simulink model "test_mpu6050"  (R2024b)
settings: Solver=FixedStepAuto  StartTime=0.0  StopTime=60  FixedStep=dt  RelTol=1e-3
model workspace (MAT data in the model file):
  dt = Simulink.Parameter
  dt.Value = 0.001
  dt.Complexity = 'real'
  dt.Dimensions = [1 1]
  dt.DataType = 'auto'
libraries: simulink x2
settings Model: ExtModeTrigDuration=2  Creator=schwmaxi  LastModifiedBy=schwmaxi
settings SolverCC: PositivePriorityOrder=on
settings OptimizationCC: BlockReduction=off  BooleanDataType=off  DefaultParameterBehavior=Inlined  EnhancedBackFolding=on  PassReuseOutputArgsAs=Individual arguments  ZeroExternalMemoryAtStartup=off  ZeroInternalMemoryAtStartup=off  MaxStackSize=200000  OptimizeBlockOrder=speed  DifferentSizesBufferReuse=on  OptimizationCustomize=off  EfficientTunableParamExpr=on
settings DebuggingCC: SaveWithParameterizedLinksMsg=none  UnderspecifiedInitializationDetection=Classic  MergeDetectMultiDrivingBlocksExec=none  SignalResolutionControl=TryResolveAllWithWarning  ParameterTunabilityLossMsg=error
settings HardwareCC: ProdBitPerPointer=32  ProdBitPerSizeT=32  ProdBitPerPtrDiffT=32  ProdLargestAtomicInteger=Long  ProdLargestAtomicFloat=Double  ProdWordSize=32  ProdLongLongMode=on  ProdHWDeviceType=ARM Compatible->ARM Cortex-A (32-bit)  UseEmbeddedCoderFeatures=off
settings ModelReferenceCC: PropagateSignalLabelsOutOfModel=off
settings RTWCC: Description=Embedded Coder  SystemTargetFile=ert.tlc  HardwareBoard=Raspberry Pi  TLCOptions="-aInlineSetEventsForThisBaseRateFcn=TLC_FALSE -aSuppressMultiTaskScheduler=TLC_FALSE  -aRateBasedStepFcn=0"  TemplateMakefile=ert_default_tmf  Toolchain=GNU GCC Embedded Linux
settings CodeAppCC: ForceParamTrailComments=on  IgnoreCustomStorageClasses=off  OperatorAnnotations=on  SimulinkDataObjDesc=on  SFDataObjDesc=on  InsertBlockDesc=on
settings ERTTargetCC: SupportNonInlinedSFcns=on  SupportVariableSizeSignals=on  ExtModeTransport=2  ExtModeStaticAlloc=on  ExtModeMexFile=ext_xcp  ExtModeIntrfLevel=Level2 - Open

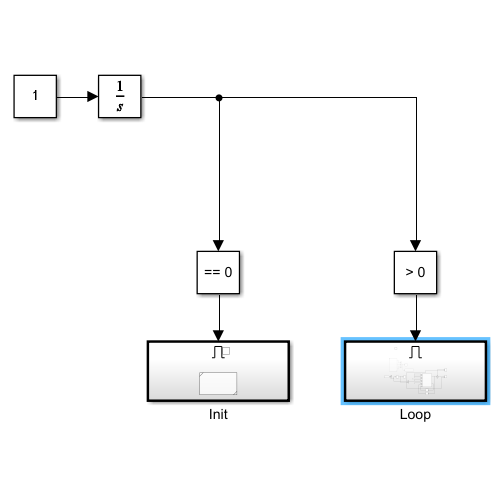
[thumbnail: Simulink's stored preview of the top-level diagram]
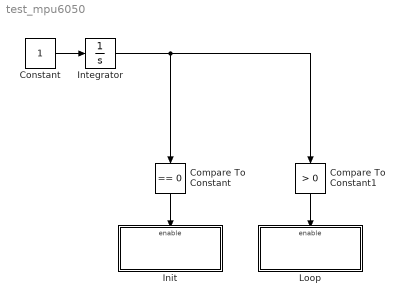
== system test_mpu6050 ==
  Compare To Constant : simulink/Logic and Bit Operations/Compare To Constant  relop===  const=0  OutDataTypeStr=boolean
  Compare To Constant1 : simulink/Logic and Bit Operations/Compare To Constant  relop=>  const=0  OutDataTypeStr=boolean
  Constant : Constant
  Init : Subsystem  TreatAsAtomicUnit=on
  Integrator : Integrator
  Loop : Subsystem  TreatAsAtomicUnit=on
  wires:
  Compare To Constant/1 -> Init/Enable
  Integrator/1 -> Compare To Constant1/1, Compare To Constant/1
  Constant/1 -> Integrator/1
  Compare To Constant1/1 -> Loop/Enable

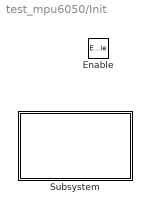
== system test_mpu6050/Init ==
  Enable : EnablePort
  Subsystem : Subsystem  ReferencedSubsystem=InitIMU

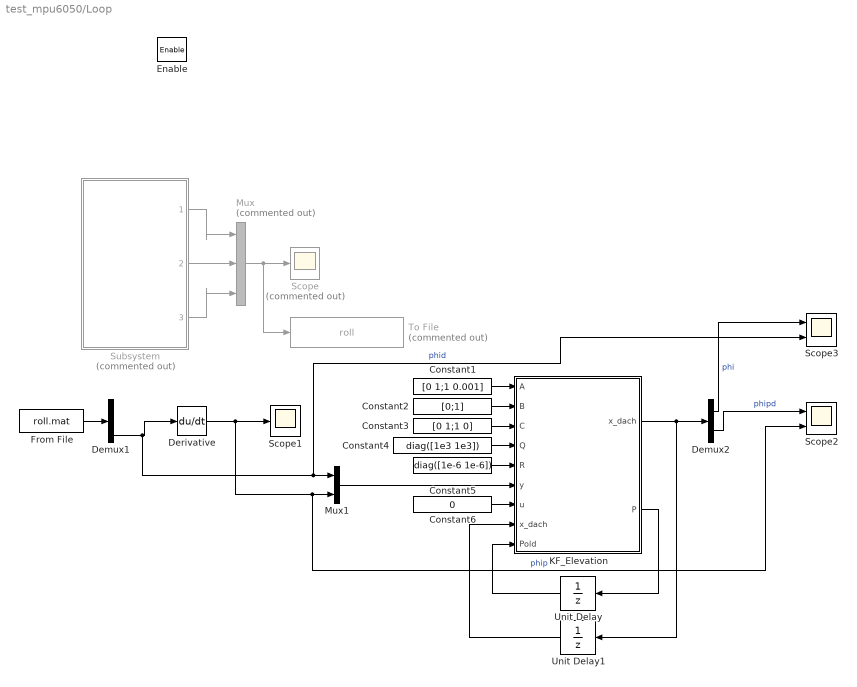
== system test_mpu6050/Loop ==
  Enable : EnablePort
  Constant1 : Constant  Value=[0 1;1 0.001]  VectorParams1D=off
  Constant2 : Constant  Value=[0;1]  VectorParams1D=off
  Constant3 : Constant  Value=[0 1;1 0]  VectorParams1D=off
  Constant4 : Constant  Value=diag([1e3 1e3])  VectorParams1D=off
  Constant5 : Constant  Value=diag([1e-6 1e-6])  VectorParams1D=off
  Constant6 : Constant  Value=0  VectorParams1D=off
  Demux1 : Demux  Outputs=3
  Demux2 : Demux  Outputs=2
  Derivative : Derivative
  From File : FromFile  FileName=roll.mat  SampleTime=0
  KF_Elevation : MATLAB Function  TreatAsAtomicUnit=on
  Mux : Mux  Commented=on  Inputs=3
  Mux1 : Mux  Inputs=2
  Scope : Scope  Commented=on
  Scope1 : Scope
  Scope2 : Scope  NumInputPorts=2
  Scope3 : Scope  NumInputPorts=2
  Subsystem : Subsystem  Commented=on  ReferencedSubsystem=IMU
  To File : ToFile  Commented=on  Filename=roll  SampleTime=0.001
  Unit Delay : UnitDelay  InitialCondition=diag([1 1e10])  SampleTime=-1  HasFrameUpgradeWarning=on
  Unit Delay1 : UnitDelay  InitialCondition=zeros(2,1)  SampleTime=-1  HasFrameUpgradeWarning=on
  wires:
  Subsystem/2 -> Mux/2
  Subsystem/1 -> Mux/1
  Subsystem/3 -> Mux/3
  Mux/1 -> To File/1, Scope/1
  KF_Elevation/1(x_dach) -> Unit Delay1/1, Demux2/1
  Constant4/1 -> KF_Elevation/4(Q)
  KF_Elevation/2(P) -> Unit Delay/1
  Constant1/1 -> KF_Elevation/1(A)
  Constant2/1 -> KF_Elevation/2(B)
  Unit Delay/1 -> KF_Elevation/9(Pold)
  Constant5/1 -> KF_Elevation/5(R)
  Constant3/1 -> KF_Elevation/3(C)
  Unit Delay1/1 -> KF_Elevation/8("x_dach ")
  From File/1 -> Demux1/1
  Demux1/3 -> Scope3/2, Mux1/1, Derivative/1  "phid"
  Derivative/1 -> Scope2/2, Mux1/2, Scope1/1  "phip"
  Demux2/2 -> Scope2/1  "phipd"
  Demux2/1 -> Scope3/1  "phi"
  Mux1/1 -> KF_Elevation/6(y)
  Constant6/1 -> KF_Elevation/7(u)

== matlab function test_mpu6050/Loop/KF_Elevation ==
  settings: updateMethod=DISCRETE
  data: A input; B input; x_dach output; C input; Q input; R input; y input; u input; x_dach input; P output; Pold input
% LQE
% DDMLTS
% Universität Augsburg
% Lehrstuhl Regelungstechnik
% F. Friedrich, 02.02.2022
function [x_dach,P]  = LQE(A,B,C,Q,R,y,u,x_dach,Pold)

% PRÄDIKTION:
% 1. Schritt: Kovarianzmatrix prädizieren:
P_pred = A * Pold * A' + Q;

% 2. Schritt: Parameterschätzung prädizieren:
x_pred = A * x_dach + B *u;

% KORREKTUR:
% 3. Schritt: Verstärkung korrigieren
K = P_pred * C' / (R + C * P_pred * C');

% 4. Schritt: Parameterschätzung korrigieren
x_dach = x_pred + K * (y - C * x_pred);

% 5. Schritt: Kovarianzmatrix korrigieren
P = (eye(size(P_pred)) - K * C) * P_pred * (eye(size(P_pred)) - K * C)' + K * R * K';

end
